simulink model "six_plus_six_AcmsteeringV09_main"  (R2014a)
settings: Solver=FixedStepDiscrete  StartTime=0.0  StopTime=10.0  FixedStep=0.0005  RelTol=1e-3
InitFcn:
  | Veh_Par_wxt
values from neighbouring files (symbols this model uses):
  acc_spdctl = [0 100]    [Veh_Par_wxt.m]
  ag_thr = ecucoder_cal(ag_thr)    [Veh_Par_wxt.m]
  B = 1.8    [Veh_Par_wxt.m]
  bra_em = 100    [Veh_Par_wxt.m]
  bra_pre_gz2 = 100/3    (= 33.3333333333)    [Veh_Par_wxt.m]
  bra_pre_gz34 = 10/3    (= 3.33333333333)    [Veh_Par_wxt.m]
  bra_pre_yd = 10/2    (= 5)    [Veh_Par_wxt.m]
  brakepre_dem_data = [0 1 2 3 4 5 6 7 8 9 10]    [Veh_Par_wxt.m]
  brakeTrq_dem_data = [0 125 251 376 502 627 753 878 1004 1129 1255]    [Veh_Par_wxt.m]
  bratrq_max = 4*1255    (= 5020)    [Veh_Par_wxt.m]
  eff_tran = 0.9    [Veh_Par_wxt.m]
  ESP_switch = ecucoder_cal(ESP_switch)    [Veh_Par_wxt.m]
  G = Mass*g    (= 15696)    [Veh_Par_wxt.m]
  kd1 = ecucoder_cal(kd1)    [Veh_Par_wxt.m]
  kd2 = 0    [Veh_Par_wxt.m]
  ki1 = ecucoder_cal(ki1)    [Veh_Par_wxt.m]
  ki2 = 1    [Veh_Par_wxt.m]
  kp1 = ecucoder_cal(kp1)    [Veh_Par_wxt.m]
  kp2 = 300    [Veh_Par_wxt.m]
  L = L1+L2    (= 2.9)    [Veh_Par_wxt.m]
  premax = 100    [Veh_Par_wxt.m]
  Radius = 0.4572/2    (= 0.2286)    [Veh_Par_wxt.m]
  RC_switch = ecucoder_cal(RC_switch)    [Veh_Par_wxt.m]
  s_opt_yi = 0.15    [Veh_Par_wxt.m]
  s_opt_zhuan = 0.8    [Veh_Par_wxt.m]
  s_opt_zhuan_add = 0.05    [Veh_Par_wxt.m]
  s_opt_zhuan_table = [0.8 0.8 0.3 0.3]    [Veh_Par_wxt.m]
  spd_map_mot = [0 499.85 999.79 1500 2000 2500 3000 3500 4000 4500 4999.8 5999.8]    [Veh_Par_wxt.m]
  spd_spdctl = [0 500]    [Veh_Par_wxt.m]
  speed_thr_park = 5/3.6/Radius*tras_ratio*30/pi    (= 464.143899364)    [Veh_Par_wxt.m]
  TCS_switch = ecucoder_cal(TCS_switch)    [Veh_Par_wxt.m]
  tras_ratio = 8    [Veh_Par_wxt.m]
  trq_map_mot = [70.5 70.012 71.154 65.797 53.917 45.159 38.073 32.685 27.48 17.133 14.949 10.07]    [Veh_Par_wxt.m]
  trqmax_yd = 70.5    [Veh_Par_wxt.m]
  trqmax_zx = 70.5    [Veh_Par_wxt.m]
  trqmaxneg = -70.5    [Veh_Par_wxt.m]
  v_gain = 0.9    [Veh_Par_wxt.m]
  v_table = [0 5 20 100]    [Veh_Par_wxt.m]
  v_thr_park = 5    [Veh_Par_wxt.m]
  zhidong_bianmazhi = [-140000 750000]    [Veh_Par_wxt.m]
  zhidong_down = -140000    [Veh_Par_wxt.m]
  zhidong_up = 750000    [Veh_Par_wxt.m]
  zhidong_youmen = [0 100]    [Veh_Par_wxt.m]
  zhuanxiang_bianmazhi = [-400000 0 400000]    [Veh_Par_wxt.m]
  zhuanxiang_down = -400000    [Veh_Par_wxt.m]
  zhuanxiang_up = 400000    [Veh_Par_wxt.m]
  zhuanxiang_youmen = [-100 0 100]    [Veh_Par_wxt.m]
undefined symbols (not defined in the file or in its folder): ecucoder_acal, guzhang_lf, guzhang_lm, guzhang_lr, guzhang_rf, guzhang_rm, guzhang_rr, myFIS
libraries: simulink x979, ec5744lib x59, fuzblock x2
(part 5 of 26)

== system six_plus_six_AcmsteeringV09_main/Data_input/7/Enabled Subsystem ==
  In2 : Inport
  Enable : EnablePort
  Data Type Conversion{,1..7} (8 alike) : DataTypeConversion
  Demux1 : Demux  Outputs=8
  MATLAB Function : MATLAB Function  TreatAsAtomicUnit=on
  MATLAB Function1 : MATLAB Function  TreatAsAtomicUnit=on
  NorthSpd_Out : Outport
  SkySpd_Out : Outport  Port=2
  wires:
  Demux1/8 -> Data Type Conversion7/1
  Demux1/7 -> Data Type Conversion6/1
  Demux1/6 -> Data Type Conversion5/1
  Demux1/5 -> Data Type Conversion4/1
  MATLAB Function1/1(y) -> SkySpd_Out/1
  MATLAB Function/1(y) -> NorthSpd_Out/1
  Demux1/1 -> Data Type Conversion/1
  Demux1/2 -> Data Type Conversion1/1
  Demux1/3 -> Data Type Conversion2/1
  Demux1/4 -> Data Type Conversion3/1
  In2/1 -> Demux1/1
  Data Type Conversion/1 -> MATLAB Function/1(data1)
  Data Type Conversion2/1 -> MATLAB Function/3(data3)
  Data Type Conversion1/1 -> MATLAB Function/2(data2)
  Data Type Conversion6/1 -> MATLAB Function1/3(data3)
  Data Type Conversion5/1 -> MATLAB Function1/2(data2)
  Data Type Conversion4/1 -> MATLAB Function1/1(data1)
  Data Type Conversion7/1 -> MATLAB Function1/4(data4)
  Data Type Conversion3/1 -> MATLAB Function/4(data4)

== system six_plus_six_AcmsteeringV09_main/Data_input/8/Enabled Subsystem ==
  In2 : Inport
  Enable : EnablePort
  Data Type Conversion{,1..7} (8 alike) : DataTypeConversion
  Demux1 : Demux  Outputs=8
  MATLAB Function : MATLAB Function  TreatAsAtomicUnit=on
  MATLAB Function1 : MATLAB Function  TreatAsAtomicUnit=on
  EastSpd_Out : Outport
  Altitude_Out : Outport  Port=2
  wires:
  In2/1 -> Demux1/1
  Demux1/4 -> Data Type Conversion3/1
  Demux1/3 -> Data Type Conversion2/1
  Demux1/2 -> Data Type Conversion1/1
  Demux1/1 -> Data Type Conversion/1
  MATLAB Function/1(y) -> EastSpd_Out/1
  MATLAB Function1/1(y) -> Altitude_Out/1
  Demux1/5 -> Data Type Conversion4/1
  Demux1/6 -> Data Type Conversion5/1
  Demux1/7 -> Data Type Conversion6/1
  Demux1/8 -> Data Type Conversion7/1
  Data Type Conversion/1 -> MATLAB Function/1(data1)
  Data Type Conversion5/1 -> MATLAB Function1/2(data2)
  Data Type Conversion2/1 -> MATLAB Function/3(data3)
  Data Type Conversion1/1 -> MATLAB Function/2(data2)
  Data Type Conversion7/1 -> MATLAB Function1/4(data4)
  Data Type Conversion4/1 -> MATLAB Function1/1(data1)
  Data Type Conversion6/1 -> MATLAB Function1/3(data3)
  Data Type Conversion3/1 -> MATLAB Function/4(data4)

== system six_plus_six_AcmsteeringV09_main/Data_input/9/Enabled Subsystem ==
  In2 : Inport
  Enable : EnablePort
  Data Type Conversion{,1..7} (8 alike) : DataTypeConversion
  Demux1 : Demux  Outputs=8
  MATLAB Function : MATLAB Function  TreatAsAtomicUnit=on
  MATLAB Function1 : MATLAB Function  TreatAsAtomicUnit=on
  Longitude_Out : Outport
  Latitude_Out : Outport  Port=2
  wires:
  Demux1/8 -> Data Type Conversion7/1
  Demux1/7 -> Data Type Conversion6/1
  Demux1/6 -> Data Type Conversion5/1
  Demux1/5 -> Data Type Conversion4/1
  MATLAB Function1/1(y) -> Latitude_Out/1
  MATLAB Function/1(y) -> Longitude_Out/1
  Demux1/1 -> Data Type Conversion/1
  Demux1/2 -> Data Type Conversion1/1
  Demux1/3 -> Data Type Conversion2/1
  Demux1/4 -> Data Type Conversion3/1
  In2/1 -> Demux1/1
  Data Type Conversion4/1 -> MATLAB Function1/1(data1)
  Data Type Conversion2/1 -> MATLAB Function/3(data3)
  Data Type Conversion1/1 -> MATLAB Function/2(data2)
  Data Type Conversion3/1 -> MATLAB Function/4(data4)
  Data Type Conversion5/1 -> MATLAB Function1/2(data2)
  Data Type Conversion6/1 -> MATLAB Function1/3(data3)
  Data Type Conversion/1 -> MATLAB Function/1(data1)
  Data Type Conversion7/1 -> MATLAB Function1/4(data4)

== system six_plus_six_AcmsteeringV09_main/Data_input/BMS1/BMS1 ==
  input : Inport
  Enable : EnablePort
  BMS1_SOC_Ad : Sum
  BMS1_SOC_Convert : DataTypeConversion  OutDataTypeStr=uint32
  BMS1_SOC_F : Gain  Gain=0.1
  BMS1_SOC_L : simulink/Logic and Bit Operations/Bitwise Operator  logicop=AND  UseBitMask=on  BitMask=65535  BitMaskRealWorld=Stored Integer
  BMS1_SOC_O : Constant  Value=0  OutDataTypeStr=single
  BMS1_SOC_S : ArithShift
  BMS1_SOC_Sub : Subsystem
  BMS1_SOC_sat : Saturate  UpperLimit=1000  LowerLimit=0
  BMS1_SOCcv : DataTypeConversion
  BMS1_SOCinput5_Ad : Sum
  BMS1_SOCinput5_C : Constant  Value=256
  BMS1_SOCinput5_P : Product
  BMS1_Sys_Status1_Ad : Sum
  BMS1_Sys_Status1_Convert : DataTypeConversion  OutDataTypeStr=uint32
  BMS1_Sys_Status1_F : Gain
  BMS1_Sys_Status1_L : simulink/Logic and Bit Operations/Bitwise Operator  logicop=AND  UseBitMask=on  BitMask=255  BitMaskRealWorld=Stored Integer
  BMS1_Sys_Status1_O : Constant  Value=0  OutDataTypeStr=single
  BMS1_Sys_Status1_S : ArithShift
  BMS1_Sys_Status1_Sub : Subsystem
  BMS1_Sys_Status1_sat : Saturate  UpperLimit=255  LowerLimit=0
  BMS1_Sys_Status1cv : DataTypeConversion
  BMS1_Sys_Status2_Ad : Sum
  BMS1_Sys_Status2_Convert : DataTypeConversion  OutDataTypeStr=uint32
  BMS1_Sys_Status2_F : Gain
  BMS1_Sys_Status2_L : simulink/Logic and Bit Operations/Bitwise Operator  logicop=AND  UseBitMask=on  BitMask=255  BitMaskRealWorld=Stored Integer
  BMS1_Sys_Status2_O : Constant  Value=0  OutDataTypeStr=single
  BMS1_Sys_Status2_S : ArithShift
  BMS1_Sys_Status2_Sub : Subsystem
  BMS1_Sys_Status2_sat : Saturate  UpperLimit=255  LowerLimit=0
  BMS1_Sys_Status2cv : DataTypeConversion
  BMS1_TotalCurrent_Ad : Sum
  BMS1_TotalCurrent_Convert : DataTypeConversion  OutDataTypeStr=uint32
  BMS1_TotalCurrent_F : Gain  Gain=0.1
  BMS1_TotalCurrent_L : simulink/Logic and Bit Operations/Bitwise Operator  logicop=AND  UseBitMask=on  BitMask=65535  BitMaskRealWorld=Stored Integer
  BMS1_TotalCurrent_O : Constant  Value=-32000  OutDataTypeStr=single
  BMS1_TotalCurrent_S : ArithShift
  BMS1_TotalCurrent_Sub : Subsystem
  BMS1_TotalCurrent_sat : Saturate  UpperLimit=3353.5  LowerLimit=-32000
  BMS1_TotalCurrentcv : DataTypeConversion
  BMS1_TotalCurrentinput3_Ad : Sum
  BMS1_TotalCurrentinput3_C : Constant  Value=256
  BMS1_TotalCurrentinput3_P : Product
  BMS1_TotalVol_Ad : Sum
  BMS1_TotalVol_Convert : DataTypeConversion  OutDataTypeStr=uint32
  BMS1_TotalVol_F : Gain  Gain=0.1
  BMS1_TotalVol_L : simulink/Logic and Bit Operations/Bitwise Operator  logicop=AND  UseBitMask=on  BitMask=65535  BitMaskRealWorld=Stored Integer
  BMS1_TotalVol_O : Constant  Value=0  OutDataTypeStr=single
  BMS1_TotalVol_S : ArithShift
  BMS1_TotalVol_Sub : Subsystem
  BMS1_TotalVol_sat : Saturate  UpperLimit=6553.5  LowerLimit=0
  BMS1_TotalVolcv : DataTypeConversion
  BMS1_TotalVolinput1_Ad : Sum
  BMS1_TotalVolinput1_C : Constant  Value=256
  BMS1_TotalVolinput1_P : Product
  Demux : Demux  Outputs=8
  BMS1_TotalVol_Out : Outport
  BMS1_TotalCurrent_Out : Outport  Port=2
  BMS1_Sys_Status2_Out : Outport  Port=3
  BMS1_Sys_Status1_Out : Outport  Port=4
  BMS1_SOC_Out : Outport  Port=5
  wires:
  BMS1_TotalVol_F/1 -> BMS1_TotalVol_Ad/1
  BMS1_TotalVol_O/1 -> BMS1_TotalVol_Ad/2
  BMS1_TotalVol_Ad/1 -> BMS1_TotalVol_sat/1
  BMS1_TotalVol_sat/1 -> BMS1_TotalVol_Out/1
  Demux/1 -> BMS1_TotalVolinput1_P/1
  BMS1_TotalVolinput1_C/1 -> BMS1_TotalVolinput1_P/2
  BMS1_TotalVolinput1_P/1 -> BMS1_TotalVolinput1_Ad/1
  Demux/2 -> BMS1_TotalVolinput1_Ad/2
  BMS1_TotalVolinput1_Ad/1 -> BMS1_TotalVol_Sub/1(In1)
  BMS1_TotalVol_Sub/1(Out1) -> BMS1_TotalVol_Convert/1
  BMS1_TotalVol_Convert/1 -> BMS1_TotalVol_L/1
  BMS1_TotalVol_L/1 -> BMS1_TotalVol_S/1
  BMS1_TotalVol_S/1 -> BMS1_TotalVolcv/1
  BMS1_TotalVolcv/1 -> BMS1_TotalVol_F/1
  BMS1_TotalCurrent_F/1 -> BMS1_TotalCurrent_Ad/1
  BMS1_TotalCurrent_O/1 -> BMS1_TotalCurrent_Ad/2
  BMS1_TotalCurrent_Ad/1 -> BMS1_TotalCurrent_sat/1
  BMS1_TotalCurrent_sat/1 -> BMS1_TotalCurrent_Out/1
  Demux/3 -> BMS1_TotalCurrentinput3_P/1
  BMS1_TotalCurrentinput3_C/1 -> BMS1_TotalCurrentinput3_P/2
  BMS1_TotalCurrentinput3_P/1 -> BMS1_TotalCurrentinput3_Ad/1
  Demux/4 -> BMS1_TotalCurrentinput3_Ad/2
  BMS1_TotalCurrentinput3_Ad/1 -> BMS1_TotalCurrent_Sub/1(In1)
  BMS1_TotalCurrent_Sub/1(Out1) -> BMS1_TotalCurrent_Convert/1
  BMS1_TotalCurrent_Convert/1 -> BMS1_TotalCurrent_L/1
  BMS1_TotalCurrent_L/1 -> BMS1_TotalCurrent_S/1
  BMS1_TotalCurrent_S/1 -> BMS1_TotalCurrentcv/1
  BMS1_TotalCurrentcv/1 -> BMS1_TotalCurrent_F/1
  BMS1_Sys_Status2_F/1 -> BMS1_Sys_Status2_Ad/1
  BMS1_Sys_Status2_O/1 -> BMS1_Sys_Status2_Ad/2
  BMS1_Sys_Status2_Ad/1 -> BMS1_Sys_Status2_sat/1
  BMS1_Sys_Status2_sat/1 -> BMS1_Sys_Status2_Out/1
  Demux/8 -> BMS1_Sys_Status2_Sub/1(In1)
  BMS1_Sys_Status2_Sub/1(Out1) -> BMS1_Sys_Status2_Convert/1
  BMS1_Sys_Status2_Convert/1 -> BMS1_Sys_Status2_L/1
  BMS1_Sys_Status2_L/1 -> BMS1_Sys_Status2_S/1
  BMS1_Sys_Status2_S/1 -> BMS1_Sys_Status2cv/1
  BMS1_Sys_Status2cv/1 -> BMS1_Sys_Status2_F/1
  BMS1_Sys_Status1_F/1 -> BMS1_Sys_Status1_Ad/1
  BMS1_Sys_Status1_O/1 -> BMS1_Sys_Status1_Ad/2
  BMS1_Sys_Status1_Ad/1 -> BMS1_Sys_Status1_sat/1
  BMS1_Sys_Status1_sat/1 -> BMS1_Sys_Status1_Out/1
  Demux/7 -> BMS1_Sys_Status1_Sub/1(In1)
  BMS1_Sys_Status1_Sub/1(Out1) -> BMS1_Sys_Status1_Convert/1
  BMS1_Sys_Status1_Convert/1 -> BMS1_Sys_Status1_L/1
  BMS1_Sys_Status1_L/1 -> BMS1_Sys_Status1_S/1
  BMS1_Sys_Status1_S/1 -> BMS1_Sys_Status1cv/1
  BMS1_Sys_Status1cv/1 -> BMS1_Sys_Status1_F/1
  BMS1_SOC_F/1 -> BMS1_SOC_Ad/1
  BMS1_SOC_O/1 -> BMS1_SOC_Ad/2
  BMS1_SOC_Ad/1 -> BMS1_SOC_sat/1
  BMS1_SOC_sat/1 -> BMS1_SOC_Out/1
  Demux/5 -> BMS1_SOCinput5_P/1
  BMS1_SOCinput5_C/1 -> BMS1_SOCinput5_P/2
  BMS1_SOCinput5_P/1 -> BMS1_SOCinput5_Ad/1
  Demux/6 -> BMS1_SOCinput5_Ad/2
  BMS1_SOCinput5_Ad/1 -> BMS1_SOC_Sub/1(In1)
  BMS1_SOC_Sub/1(Out1) -> BMS1_SOC_Convert/1
  BMS1_SOC_Convert/1 -> BMS1_SOC_L/1
  BMS1_SOC_L/1 -> BMS1_SOC_S/1
  BMS1_SOC_S/1 -> BMS1_SOCcv/1
  BMS1_SOCcv/1 -> BMS1_SOC_F/1
  input/1 -> Demux/1

== system six_plus_six_AcmsteeringV09_main/Data_input/BMS1-2/BMS1 ==
  input : Inport
  Enable : EnablePort
  BMS1_SOC_Ad : Sum
  BMS1_SOC_Convert : DataTypeConversion  OutDataTypeStr=uint32
  BMS1_SOC_F : Gain  Gain=0.1
  BMS1_SOC_L : simulink/Logic and Bit Operations/Bitwise Operator  logicop=AND  UseBitMask=on  BitMask=65535  BitMaskRealWorld=Stored Integer
  BMS1_SOC_O : Constant  Value=0  OutDataTypeStr=single
  BMS1_SOC_S : ArithShift
  BMS1_SOC_Sub : Subsystem
  BMS1_SOC_sat : Saturate  UpperLimit=1000  LowerLimit=0
  BMS1_SOCcv : DataTypeConversion
  BMS1_SOCinput5_Ad : Sum
  BMS1_SOCinput5_C : Constant  Value=256
  BMS1_SOCinput5_P : Product
  BMS1_Sys_Status1_Ad : Sum
  BMS1_Sys_Status1_Convert : DataTypeConversion  OutDataTypeStr=uint32
  BMS1_Sys_Status1_F : Gain
  BMS1_Sys_Status1_L : simulink/Logic and Bit Operations/Bitwise Operator  logicop=AND  UseBitMask=on  BitMask=255  BitMaskRealWorld=Stored Integer
  BMS1_Sys_Status1_O : Constant  Value=0  OutDataTypeStr=single
  BMS1_Sys_Status1_S : ArithShift
  BMS1_Sys_Status1_Sub : Subsystem
  BMS1_Sys_Status1_sat : Saturate  UpperLimit=255  LowerLimit=0
  BMS1_Sys_Status1cv : DataTypeConversion
  BMS1_Sys_Status2_Ad : Sum
  BMS1_Sys_Status2_Convert : DataTypeConversion  OutDataTypeStr=uint32
  BMS1_Sys_Status2_F : Gain
  BMS1_Sys_Status2_L : simulink/Logic and Bit Operations/Bitwise Operator  logicop=AND  UseBitMask=on  BitMask=255  BitMaskRealWorld=Stored Integer
  BMS1_Sys_Status2_O : Constant  Value=0  OutDataTypeStr=single
  BMS1_Sys_Status2_S : ArithShift
  BMS1_Sys_Status2_Sub : Subsystem
  BMS1_Sys_Status2_sat : Saturate  UpperLimit=255  LowerLimit=0
  BMS1_Sys_Status2cv : DataTypeConversion
  BMS1_TotalCurrent_Ad : Sum
  BMS1_TotalCurrent_Convert : DataTypeConversion  OutDataTypeStr=uint32
  BMS1_TotalCurrent_F : Gain  Gain=0.1
  BMS1_TotalCurrent_L : simulink/Logic and Bit Operations/Bitwise Operator  logicop=AND  UseBitMask=on  BitMask=65535  BitMaskRealWorld=Stored Integer
  BMS1_TotalCurrent_O : Constant  Value=-32000  OutDataTypeStr=single
  BMS1_TotalCurrent_S : ArithShift
  BMS1_TotalCurrent_Sub : Subsystem
  BMS1_TotalCurrent_sat : Saturate  UpperLimit=3353.5  LowerLimit=-32000
  BMS1_TotalCurrentcv : DataTypeConversion
  BMS1_TotalCurrentinput3_Ad : Sum
  BMS1_TotalCurrentinput3_C : Constant  Value=256
  BMS1_TotalCurrentinput3_P : Product
  BMS1_TotalVol_Ad : Sum
  BMS1_TotalVol_Convert : DataTypeConversion  OutDataTypeStr=uint32
  BMS1_TotalVol_F : Gain  Gain=0.1
  BMS1_TotalVol_L : simulink/Logic and Bit Operations/Bitwise Operator  logicop=AND  UseBitMask=on  BitMask=65535  BitMaskRealWorld=Stored Integer
  BMS1_TotalVol_O : Constant  Value=0  OutDataTypeStr=single
  BMS1_TotalVol_S : ArithShift
  BMS1_TotalVol_Sub : Subsystem
  BMS1_TotalVol_sat : Saturate  UpperLimit=6553.5  LowerLimit=0
  BMS1_TotalVolcv : DataTypeConversion
  BMS1_TotalVolinput1_Ad : Sum
  BMS1_TotalVolinput1_C : Constant  Value=256
  BMS1_TotalVolinput1_P : Product
  Demux : Demux  Outputs=8
  BMS1_TotalVol_Out : Outport
  BMS1_TotalCurrent_Out : Outport  Port=2
  BMS1_Sys_Status2_Out : Outport  Port=3
  BMS1_Sys_Status1_Out : Outport  Port=4
  BMS1_SOC_Out : Outport  Port=5
  wires:
  BMS1_TotalVol_F/1 -> BMS1_TotalVol_Ad/1
  BMS1_TotalVol_O/1 -> BMS1_TotalVol_Ad/2
  BMS1_TotalVol_Ad/1 -> BMS1_TotalVol_sat/1
  BMS1_TotalVol_sat/1 -> BMS1_TotalVol_Out/1
  Demux/1 -> BMS1_TotalVolinput1_P/1
  BMS1_TotalVolinput1_C/1 -> BMS1_TotalVolinput1_P/2
  BMS1_TotalVolinput1_P/1 -> BMS1_TotalVolinput1_Ad/1
  Demux/2 -> BMS1_TotalVolinput1_Ad/2
  BMS1_TotalVolinput1_Ad/1 -> BMS1_TotalVol_Sub/1(In1)
  BMS1_TotalVol_Sub/1(Out1) -> BMS1_TotalVol_Convert/1
  BMS1_TotalVol_Convert/1 -> BMS1_TotalVol_L/1
  BMS1_TotalVol_L/1 -> BMS1_TotalVol_S/1
  BMS1_TotalVol_S/1 -> BMS1_TotalVolcv/1
  BMS1_TotalVolcv/1 -> BMS1_TotalVol_F/1
  BMS1_TotalCurrent_F/1 -> BMS1_TotalCurrent_Ad/1
  BMS1_TotalCurrent_O/1 -> BMS1_TotalCurrent_Ad/2
  BMS1_TotalCurrent_Ad/1 -> BMS1_TotalCurrent_sat/1
  BMS1_TotalCurrent_sat/1 -> BMS1_TotalCurrent_Out/1
  Demux/3 -> BMS1_TotalCurrentinput3_P/1
  BMS1_TotalCurrentinput3_C/1 -> BMS1_TotalCurrentinput3_P/2
  BMS1_TotalCurrentinput3_P/1 -> BMS1_TotalCurrentinput3_Ad/1
  Demux/4 -> BMS1_TotalCurrentinput3_Ad/2
  BMS1_TotalCurrentinput3_Ad/1 -> BMS1_TotalCurrent_Sub/1(In1)
  BMS1_TotalCurrent_Sub/1(Out1) -> BMS1_TotalCurrent_Convert/1
  BMS1_TotalCurrent_Convert/1 -> BMS1_TotalCurrent_L/1
  BMS1_TotalCurrent_L/1 -> BMS1_TotalCurrent_S/1
  BMS1_TotalCurrent_S/1 -> BMS1_TotalCurrentcv/1
  BMS1_TotalCurrentcv/1 -> BMS1_TotalCurrent_F/1
  BMS1_Sys_Status2_F/1 -> BMS1_Sys_Status2_Ad/1
  BMS1_Sys_Status2_O/1 -> BMS1_Sys_Status2_Ad/2
  BMS1_Sys_Status2_Ad/1 -> BMS1_Sys_Status2_sat/1
  BMS1_Sys_Status2_sat/1 -> BMS1_Sys_Status2_Out/1
  Demux/8 -> BMS1_Sys_Status2_Sub/1(In1)
  BMS1_Sys_Status2_Sub/1(Out1) -> BMS1_Sys_Status2_Convert/1
  BMS1_Sys_Status2_Convert/1 -> BMS1_Sys_Status2_L/1
  BMS1_Sys_Status2_L/1 -> BMS1_Sys_Status2_S/1
  BMS1_Sys_Status2_S/1 -> BMS1_Sys_Status2cv/1
  BMS1_Sys_Status2cv/1 -> BMS1_Sys_Status2_F/1
  BMS1_Sys_Status1_F/1 -> BMS1_Sys_Status1_Ad/1
  BMS1_Sys_Status1_O/1 -> BMS1_Sys_Status1_Ad/2
  BMS1_Sys_Status1_Ad/1 -> BMS1_Sys_Status1_sat/1
  BMS1_Sys_Status1_sat/1 -> BMS1_Sys_Status1_Out/1
  Demux/7 -> BMS1_Sys_Status1_Sub/1(In1)
  BMS1_Sys_Status1_Sub/1(Out1) -> BMS1_Sys_Status1_Convert/1
  BMS1_Sys_Status1_Convert/1 -> BMS1_Sys_Status1_L/1
  BMS1_Sys_Status1_L/1 -> BMS1_Sys_Status1_S/1
  BMS1_Sys_Status1_S/1 -> BMS1_Sys_Status1cv/1
  BMS1_Sys_Status1cv/1 -> BMS1_Sys_Status1_F/1
  BMS1_SOC_F/1 -> BMS1_SOC_Ad/1
  BMS1_SOC_O/1 -> BMS1_SOC_Ad/2
  BMS1_SOC_Ad/1 -> BMS1_SOC_sat/1
  BMS1_SOC_sat/1 -> BMS1_SOC_Out/1
  Demux/5 -> BMS1_SOCinput5_P/1
  BMS1_SOCinput5_C/1 -> BMS1_SOCinput5_P/2
  BMS1_SOCinput5_P/1 -> BMS1_SOCinput5_Ad/1
  Demux/6 -> BMS1_SOCinput5_Ad/2
  BMS1_SOCinput5_Ad/1 -> BMS1_SOC_Sub/1(In1)
  BMS1_SOC_Sub/1(Out1) -> BMS1_SOC_Convert/1
  BMS1_SOC_Convert/1 -> BMS1_SOC_L/1
  BMS1_SOC_L/1 -> BMS1_SOC_S/1
  BMS1_SOC_S/1 -> BMS1_SOCcv/1
  BMS1_SOCcv/1 -> BMS1_SOC_F/1
  input/1 -> Demux/1

== system six_plus_six_AcmsteeringV09_main/Data_input/BMS1_1/BMS1 ==
  input : Inport
  Enable : EnablePort
  BMS1_SOC_Ad : Sum
  BMS1_SOC_Convert : DataTypeConversion  OutDataTypeStr=uint32
  BMS1_SOC_F : Gain  Gain=0.1
  BMS1_SOC_L : simulink/Logic and Bit Operations/Bitwise Operator  logicop=AND  UseBitMask=on  BitMask=65535  BitMaskRealWorld=Stored Integer
  BMS1_SOC_O : Constant  Value=0  OutDataTypeStr=single
  BMS1_SOC_S : ArithShift
  BMS1_SOC_Sub : Subsystem
  BMS1_SOC_sat : Saturate  UpperLimit=1000  LowerLimit=0
  BMS1_SOCcv : DataTypeConversion
  BMS1_SOCinput5_Ad : Sum
  BMS1_SOCinput5_C : Constant  Value=256
  BMS1_SOCinput5_P : Product
  BMS1_Sys_Status1_Ad : Sum
  BMS1_Sys_Status1_Convert : DataTypeConversion  OutDataTypeStr=uint32
  BMS1_Sys_Status1_F : Gain
  BMS1_Sys_Status1_L : simulink/Logic and Bit Operations/Bitwise Operator  logicop=AND  UseBitMask=on  BitMask=255  BitMaskRealWorld=Stored Integer
  BMS1_Sys_Status1_O : Constant  Value=0  OutDataTypeStr=single
  BMS1_Sys_Status1_S : ArithShift
  BMS1_Sys_Status1_Sub : Subsystem
  BMS1_Sys_Status1_sat : Saturate  UpperLimit=255  LowerLimit=0
  BMS1_Sys_Status1cv : DataTypeConversion
  BMS1_Sys_Status2_Ad : Sum
  BMS1_Sys_Status2_Convert : DataTypeConversion  OutDataTypeStr=uint32
  BMS1_Sys_Status2_F : Gain
  BMS1_Sys_Status2_L : simulink/Logic and Bit Operations/Bitwise Operator  logicop=AND  UseBitMask=on  BitMask=255  BitMaskRealWorld=Stored Integer
  BMS1_Sys_Status2_O : Constant  Value=0  OutDataTypeStr=single
  BMS1_Sys_Status2_S : ArithShift
  BMS1_Sys_Status2_Sub : Subsystem
  BMS1_Sys_Status2_sat : Saturate  UpperLimit=255  LowerLimit=0
  BMS1_Sys_Status2cv : DataTypeConversion
  BMS1_TotalCurrent_Ad : Sum
  BMS1_TotalCurrent_Convert : DataTypeConversion  OutDataTypeStr=uint32
  BMS1_TotalCurrent_F : Gain  Gain=0.1
  BMS1_TotalCurrent_L : simulink/Logic and Bit Operations/Bitwise Operator  logicop=AND  UseBitMask=on  BitMask=65535  BitMaskRealWorld=Stored Integer
  BMS1_TotalCurrent_O : Constant  Value=-32000  OutDataTypeStr=single
  BMS1_TotalCurrent_S : ArithShift
  BMS1_TotalCurrent_Sub : Subsystem
  BMS1_TotalCurrent_sat : Saturate  UpperLimit=3353.5  LowerLimit=-32000
  BMS1_TotalCurrentcv : DataTypeConversion
  BMS1_TotalCurrentinput3_Ad : Sum
  BMS1_TotalCurrentinput3_C : Constant  Value=256
  BMS1_TotalCurrentinput3_P : Product
  BMS1_TotalVol_Ad : Sum
  BMS1_TotalVol_Convert : DataTypeConversion  OutDataTypeStr=uint32
  BMS1_TotalVol_F : Gain  Gain=0.1
  BMS1_TotalVol_L : simulink/Logic and Bit Operations/Bitwise Operator  logicop=AND  UseBitMask=on  BitMask=65535  BitMaskRealWorld=Stored Integer
  BMS1_TotalVol_O : Constant  Value=0  OutDataTypeStr=single
  BMS1_TotalVol_S : ArithShift
  BMS1_TotalVol_Sub : Subsystem
  BMS1_TotalVol_sat : Saturate  UpperLimit=6553.5  LowerLimit=0
  BMS1_TotalVolcv : DataTypeConversion
  BMS1_TotalVolinput1_Ad : Sum
  BMS1_TotalVolinput1_C : Constant  Value=256
  BMS1_TotalVolinput1_P : Product
  Demux : Demux  Outputs=8
  BMS1_TotalVol_Out : Outport
  BMS1_TotalCurrent_Out : Outport  Port=2
  BMS1_Sys_Status2_Out : Outport  Port=3
  BMS1_Sys_Status1_Out : Outport  Port=4
  BMS1_SOC_Out : Outport  Port=5
  wires:
  BMS1_TotalVol_F/1 -> BMS1_TotalVol_Ad/1
  BMS1_TotalVol_O/1 -> BMS1_TotalVol_Ad/2
  BMS1_TotalVol_Ad/1 -> BMS1_TotalVol_sat/1
  BMS1_TotalVol_sat/1 -> BMS1_TotalVol_Out/1
  Demux/1 -> BMS1_TotalVolinput1_P/1
  BMS1_TotalVolinput1_C/1 -> BMS1_TotalVolinput1_P/2
  BMS1_TotalVolinput1_P/1 -> BMS1_TotalVolinput1_Ad/1
  Demux/2 -> BMS1_TotalVolinput1_Ad/2
  BMS1_TotalVolinput1_Ad/1 -> BMS1_TotalVol_Sub/1(In1)
  BMS1_TotalVol_Sub/1(Out1) -> BMS1_TotalVol_Convert/1
  BMS1_TotalVol_Convert/1 -> BMS1_TotalVol_L/1
  BMS1_TotalVol_L/1 -> BMS1_TotalVol_S/1
  BMS1_TotalVol_S/1 -> BMS1_TotalVolcv/1
  BMS1_TotalVolcv/1 -> BMS1_TotalVol_F/1
  BMS1_TotalCurrent_F/1 -> BMS1_TotalCurrent_Ad/1
  BMS1_TotalCurrent_O/1 -> BMS1_TotalCurrent_Ad/2
  BMS1_TotalCurrent_Ad/1 -> BMS1_TotalCurrent_sat/1
  BMS1_TotalCurrent_sat/1 -> BMS1_TotalCurrent_Out/1
  Demux/3 -> BMS1_TotalCurrentinput3_P/1
  BMS1_TotalCurrentinput3_C/1 -> BMS1_TotalCurrentinput3_P/2
  BMS1_TotalCurrentinput3_P/1 -> BMS1_TotalCurrentinput3_Ad/1
  Demux/4 -> BMS1_TotalCurrentinput3_Ad/2
  BMS1_TotalCurrentinput3_Ad/1 -> BMS1_TotalCurrent_Sub/1(In1)
  BMS1_TotalCurrent_Sub/1(Out1) -> BMS1_TotalCurrent_Convert/1
  BMS1_TotalCurrent_Convert/1 -> BMS1_TotalCurrent_L/1
  BMS1_TotalCurrent_L/1 -> BMS1_TotalCurrent_S/1
  BMS1_TotalCurrent_S/1 -> BMS1_TotalCurrentcv/1
  BMS1_TotalCurrentcv/1 -> BMS1_TotalCurrent_F/1
  BMS1_Sys_Status2_F/1 -> BMS1_Sys_Status2_Ad/1
  BMS1_Sys_Status2_O/1 -> BMS1_Sys_Status2_Ad/2
  BMS1_Sys_Status2_Ad/1 -> BMS1_Sys_Status2_sat/1
  BMS1_Sys_Status2_sat/1 -> BMS1_Sys_Status2_Out/1
  Demux/8 -> BMS1_Sys_Status2_Sub/1(In1)
  BMS1_Sys_Status2_Sub/1(Out1) -> BMS1_Sys_Status2_Convert/1
  BMS1_Sys_Status2_Convert/1 -> BMS1_Sys_Status2_L/1
  BMS1_Sys_Status2_L/1 -> BMS1_Sys_Status2_S/1
  BMS1_Sys_Status2_S/1 -> BMS1_Sys_Status2cv/1
  BMS1_Sys_Status2cv/1 -> BMS1_Sys_Status2_F/1
  BMS1_Sys_Status1_F/1 -> BMS1_Sys_Status1_Ad/1
  BMS1_Sys_Status1_O/1 -> BMS1_Sys_Status1_Ad/2
  BMS1_Sys_Status1_Ad/1 -> BMS1_Sys_Status1_sat/1
  BMS1_Sys_Status1_sat/1 -> BMS1_Sys_Status1_Out/1
  Demux/7 -> BMS1_Sys_Status1_Sub/1(In1)
  BMS1_Sys_Status1_Sub/1(Out1) -> BMS1_Sys_Status1_Convert/1
  BMS1_Sys_Status1_Convert/1 -> BMS1_Sys_Status1_L/1
  BMS1_Sys_Status1_L/1 -> BMS1_Sys_Status1_S/1
  BMS1_Sys_Status1_S/1 -> BMS1_Sys_Status1cv/1
  BMS1_Sys_Status1cv/1 -> BMS1_Sys_Status1_F/1
  BMS1_SOC_F/1 -> BMS1_SOC_Ad/1
  BMS1_SOC_O/1 -> BMS1_SOC_Ad/2
  BMS1_SOC_Ad/1 -> BMS1_SOC_sat/1
  BMS1_SOC_sat/1 -> BMS1_SOC_Out/1
  Demux/5 -> BMS1_SOCinput5_P/1
  BMS1_SOCinput5_C/1 -> BMS1_SOCinput5_P/2
  BMS1_SOCinput5_P/1 -> BMS1_SOCinput5_Ad/1
  Demux/6 -> BMS1_SOCinput5_Ad/2
  BMS1_SOCinput5_Ad/1 -> BMS1_SOC_Sub/1(In1)
  BMS1_SOC_Sub/1(Out1) -> BMS1_SOC_Convert/1
  BMS1_SOC_Convert/1 -> BMS1_SOC_L/1
  BMS1_SOC_L/1 -> BMS1_SOC_S/1
  BMS1_SOC_S/1 -> BMS1_SOCcv/1
  BMS1_SOCcv/1 -> BMS1_SOC_F/1
  input/1 -> Demux/1

== system six_plus_six_AcmsteeringV09_main/Data_input/BMS2/BMS2 ==
  input : Inport
  Enable : EnablePort
  BMS2_HighSingleVol_Ad : Sum
  BMS2_HighSingleVol_Convert : DataTypeConversion  OutDataTypeStr=uint32
  BMS2_HighSingleVol_F : Gain
  BMS2_HighSingleVol_L : simulink/Logic and Bit Operations/Bitwise Operator  logicop=AND  UseBitMask=on  BitMask=65535  BitMaskRealWorld=Stored Integer
  BMS2_HighSingleVol_O : Constant  Value=0  OutDataTypeStr=single
  BMS2_HighSingleVol_S : ArithShift
  BMS2_HighSingleVol_Sub : Subsystem
  BMS2_HighSingleVol_sat : Saturate  UpperLimit=10  LowerLimit=0
  BMS2_HighSingleVolcv : DataTypeConversion
  BMS2_HighSingleVolinput1_Ad : Sum
  BMS2_HighSingleVolinput1_C : Constant  Value=256
  BMS2_HighSingleVolinput1_P : Product
  BMS2_LowSingleVol_Ad : Sum
  BMS2_LowSingleVol_Convert : DataTypeConversion  OutDataTypeStr=uint32
  BMS2_LowSingleVol_F : Gain
  BMS2_LowSingleVol_L : simulink/Logic and Bit Operations/Bitwise Operator  logicop=AND  UseBitMask=on  BitMask=65535  BitMaskRealWorld=Stored Integer
  BMS2_LowSingleVol_O : Constant  Value=0  OutDataTypeStr=single
  BMS2_LowSingleVol_S : ArithShift
  BMS2_LowSingleVol_Sub : Subsystem
  BMS2_LowSingleVol_sat : Saturate  UpperLimit=65535  LowerLimit=0
  BMS2_LowSingleVolcv : DataTypeConversion
  BMS2_LowSingleVolinput3_Ad : Sum
  BMS2_LowSingleVolinput3_C : Constant  Value=256
  BMS2_LowSingleVolinput3_P : Product
  Demux : Demux  Outputs=8
  BMS2_LowSingleVol_Out : Outport
  BMS2_HighSingleVol_Out : Outport  Port=2
  wires:
  BMS2_LowSingleVol_F/1 -> BMS2_LowSingleVol_Ad/1
  BMS2_LowSingleVol_O/1 -> BMS2_LowSingleVol_Ad/2
  BMS2_LowSingleVol_Ad/1 -> BMS2_LowSingleVol_sat/1
  BMS2_LowSingleVol_sat/1 -> BMS2_LowSingleVol_Out/1
  Demux/3 -> BMS2_LowSingleVolinput3_P/1
  BMS2_LowSingleVolinput3_C/1 -> BMS2_LowSingleVolinput3_P/2
  BMS2_LowSingleVolinput3_P/1 -> BMS2_LowSingleVolinput3_Ad/1
  Demux/4 -> BMS2_LowSingleVolinput3_Ad/2
  BMS2_LowSingleVolinput3_Ad/1 -> BMS2_LowSingleVol_Sub/1(In1)
  BMS2_LowSingleVol_Sub/1(Out1) -> BMS2_LowSingleVol_Convert/1
  BMS2_LowSingleVol_Convert/1 -> BMS2_LowSingleVol_L/1
  BMS2_LowSingleVol_L/1 -> BMS2_LowSingleVol_S/1
  BMS2_LowSingleVol_S/1 -> BMS2_LowSingleVolcv/1
  BMS2_LowSingleVolcv/1 -> BMS2_LowSingleVol_F/1
  BMS2_HighSingleVol_F/1 -> BMS2_HighSingleVol_Ad/1
  BMS2_HighSingleVol_O/1 -> BMS2_HighSingleVol_Ad/2
  BMS2_HighSingleVol_Ad/1 -> BMS2_HighSingleVol_sat/1
  BMS2_HighSingleVol_sat/1 -> BMS2_HighSingleVol_Out/1
  Demux/1 -> BMS2_HighSingleVolinput1_P/1
  BMS2_HighSingleVolinput1_C/1 -> BMS2_HighSingleVolinput1_P/2
  BMS2_HighSingleVolinput1_P/1 -> BMS2_HighSingleVolinput1_Ad/1
  Demux/2 -> BMS2_HighSingleVolinput1_Ad/2
  BMS2_HighSingleVolinput1_Ad/1 -> BMS2_HighSingleVol_Sub/1(In1)
  BMS2_HighSingleVol_Sub/1(Out1) -> BMS2_HighSingleVol_Convert/1
  BMS2_HighSingleVol_Convert/1 -> BMS2_HighSingleVol_L/1
  BMS2_HighSingleVol_L/1 -> BMS2_HighSingleVol_S/1
  BMS2_HighSingleVol_S/1 -> BMS2_HighSingleVolcv/1
  BMS2_HighSingleVolcv/1 -> BMS2_HighSingleVol_F/1
  input/1 -> Demux/1

== system six_plus_six_AcmsteeringV09_main/Data_input/BMS2_1/BMS2 ==
  input : Inport
  Enable : EnablePort
  BMS2_HighSingleVol_Ad : Sum
  BMS2_HighSingleVol_Convert : DataTypeConversion  OutDataTypeStr=uint32
  BMS2_HighSingleVol_F : Gain
  BMS2_HighSingleVol_L : simulink/Logic and Bit Operations/Bitwise Operator  logicop=AND  UseBitMask=on  BitMask=65535  BitMaskRealWorld=Stored Integer
  BMS2_HighSingleVol_O : Constant  Value=0  OutDataTypeStr=single
  BMS2_HighSingleVol_S : ArithShift
  BMS2_HighSingleVol_Sub : Subsystem
  BMS2_HighSingleVol_sat : Saturate  UpperLimit=10  LowerLimit=0
  BMS2_HighSingleVolcv : DataTypeConversion
  BMS2_HighSingleVolinput1_Ad : Sum
  BMS2_HighSingleVolinput1_C : Constant  Value=256
  BMS2_HighSingleVolinput1_P : Product
  BMS2_LowSingleVol_Ad : Sum
  BMS2_LowSingleVol_Convert : DataTypeConversion  OutDataTypeStr=uint32
  BMS2_LowSingleVol_F : Gain
  BMS2_LowSingleVol_L : simulink/Logic and Bit Operations/Bitwise Operator  logicop=AND  UseBitMask=on  BitMask=65535  BitMaskRealWorld=Stored Integer
  BMS2_LowSingleVol_O : Constant  Value=0  OutDataTypeStr=single
  BMS2_LowSingleVol_S : ArithShift
  BMS2_LowSingleVol_Sub : Subsystem
  BMS2_LowSingleVol_sat : Saturate  UpperLimit=65535  LowerLimit=0
  BMS2_LowSingleVolcv : DataTypeConversion
  BMS2_LowSingleVolinput3_Ad : Sum
  BMS2_LowSingleVolinput3_C : Constant  Value=256
  BMS2_LowSingleVolinput3_P : Product
  Demux : Demux  Outputs=8
  BMS2_LowSingleVol_Out : Outport
  BMS2_HighSingleVol_Out : Outport  Port=2
  wires:
  BMS2_LowSingleVol_F/1 -> BMS2_LowSingleVol_Ad/1
  BMS2_LowSingleVol_O/1 -> BMS2_LowSingleVol_Ad/2
  BMS2_LowSingleVol_Ad/1 -> BMS2_LowSingleVol_sat/1
  BMS2_LowSingleVol_sat/1 -> BMS2_LowSingleVol_Out/1
  Demux/3 -> BMS2_LowSingleVolinput3_P/1
  BMS2_LowSingleVolinput3_C/1 -> BMS2_LowSingleVolinput3_P/2
  BMS2_LowSingleVolinput3_P/1 -> BMS2_LowSingleVolinput3_Ad/1
  Demux/4 -> BMS2_LowSingleVolinput3_Ad/2
  BMS2_LowSingleVolinput3_Ad/1 -> BMS2_LowSingleVol_Sub/1(In1)
  BMS2_LowSingleVol_Sub/1(Out1) -> BMS2_LowSingleVol_Convert/1
  BMS2_LowSingleVol_Convert/1 -> BMS2_LowSingleVol_L/1
  BMS2_LowSingleVol_L/1 -> BMS2_LowSingleVol_S/1
  BMS2_LowSingleVol_S/1 -> BMS2_LowSingleVolcv/1
  BMS2_LowSingleVolcv/1 -> BMS2_LowSingleVol_F/1
  BMS2_HighSingleVol_F/1 -> BMS2_HighSingleVol_Ad/1
  BMS2_HighSingleVol_O/1 -> BMS2_HighSingleVol_Ad/2
  BMS2_HighSingleVol_Ad/1 -> BMS2_HighSingleVol_sat/1
  BMS2_HighSingleVol_sat/1 -> BMS2_HighSingleVol_Out/1
  Demux/1 -> BMS2_HighSingleVolinput1_P/1
  BMS2_HighSingleVolinput1_C/1 -> BMS2_HighSingleVolinput1_P/2
  BMS2_HighSingleVolinput1_P/1 -> BMS2_HighSingleVolinput1_Ad/1
  Demux/2 -> BMS2_HighSingleVolinput1_Ad/2
  BMS2_HighSingleVolinput1_Ad/1 -> BMS2_HighSingleVol_Sub/1(In1)
  BMS2_HighSingleVol_Sub/1(Out1) -> BMS2_HighSingleVol_Convert/1
  BMS2_HighSingleVol_Convert/1 -> BMS2_HighSingleVol_L/1
  BMS2_HighSingleVol_L/1 -> BMS2_HighSingleVol_S/1
  BMS2_HighSingleVol_S/1 -> BMS2_HighSingleVolcv/1
  BMS2_HighSingleVolcv/1 -> BMS2_HighSingleVol_F/1
  input/1 -> Demux/1

== system six_plus_six_AcmsteeringV09_main/Data_input/BMS2_2/BMS2 ==
  input : Inport
  Enable : EnablePort
  BMS2_HighSingleVol_Ad : Sum
  BMS2_HighSingleVol_Convert : DataTypeConversion  OutDataTypeStr=uint32
  BMS2_HighSingleVol_F : Gain
  BMS2_HighSingleVol_L : simulink/Logic and Bit Operations/Bitwise Operator  logicop=AND  UseBitMask=on  BitMask=65535  BitMaskRealWorld=Stored Integer
  BMS2_HighSingleVol_O : Constant  Value=0  OutDataTypeStr=single
  BMS2_HighSingleVol_S : ArithShift
  BMS2_HighSingleVol_Sub : Subsystem
  BMS2_HighSingleVol_sat : Saturate  UpperLimit=10  LowerLimit=0
  BMS2_HighSingleVolcv : DataTypeConversion
  BMS2_HighSingleVolinput1_Ad : Sum
  BMS2_HighSingleVolinput1_C : Constant  Value=256
  BMS2_HighSingleVolinput1_P : Product
  BMS2_LowSingleVol_Ad : Sum
  BMS2_LowSingleVol_Convert : DataTypeConversion  OutDataTypeStr=uint32
  BMS2_LowSingleVol_F : Gain
  BMS2_LowSingleVol_L : simulink/Logic and Bit Operations/Bitwise Operator  logicop=AND  UseBitMask=on  BitMask=65535  BitMaskRealWorld=Stored Integer
  BMS2_LowSingleVol_O : Constant  Value=0  OutDataTypeStr=single
  BMS2_LowSingleVol_S : ArithShift
  BMS2_LowSingleVol_Sub : Subsystem
  BMS2_LowSingleVol_sat : Saturate  UpperLimit=65535  LowerLimit=0
  BMS2_LowSingleVolcv : DataTypeConversion
  BMS2_LowSingleVolinput3_Ad : Sum
  BMS2_LowSingleVolinput3_C : Constant  Value=256
  BMS2_LowSingleVolinput3_P : Product
  Demux : Demux  Outputs=8
  BMS2_LowSingleVol_Out : Outport
  BMS2_HighSingleVol_Out : Outport  Port=2
  wires:
  BMS2_LowSingleVol_F/1 -> BMS2_LowSingleVol_Ad/1
  BMS2_LowSingleVol_O/1 -> BMS2_LowSingleVol_Ad/2
  BMS2_LowSingleVol_Ad/1 -> BMS2_LowSingleVol_sat/1
  BMS2_LowSingleVol_sat/1 -> BMS2_LowSingleVol_Out/1
  Demux/3 -> BMS2_LowSingleVolinput3_P/1
  BMS2_LowSingleVolinput3_C/1 -> BMS2_LowSingleVolinput3_P/2
  BMS2_LowSingleVolinput3_P/1 -> BMS2_LowSingleVolinput3_Ad/1
  Demux/4 -> BMS2_LowSingleVolinput3_Ad/2
  BMS2_LowSingleVolinput3_Ad/1 -> BMS2_LowSingleVol_Sub/1(In1)
  BMS2_LowSingleVol_Sub/1(Out1) -> BMS2_LowSingleVol_Convert/1
  BMS2_LowSingleVol_Convert/1 -> BMS2_LowSingleVol_L/1
  BMS2_LowSingleVol_L/1 -> BMS2_LowSingleVol_S/1
  BMS2_LowSingleVol_S/1 -> BMS2_LowSingleVolcv/1
  BMS2_LowSingleVolcv/1 -> BMS2_LowSingleVol_F/1
  BMS2_HighSingleVol_F/1 -> BMS2_HighSingleVol_Ad/1
  BMS2_HighSingleVol_O/1 -> BMS2_HighSingleVol_Ad/2
  BMS2_HighSingleVol_Ad/1 -> BMS2_HighSingleVol_sat/1
  BMS2_HighSingleVol_sat/1 -> BMS2_HighSingleVol_Out/1
  Demux/1 -> BMS2_HighSingleVolinput1_P/1
  BMS2_HighSingleVolinput1_C/1 -> BMS2_HighSingleVolinput1_P/2
  BMS2_HighSingleVolinput1_P/1 -> BMS2_HighSingleVolinput1_Ad/1
  Demux/2 -> BMS2_HighSingleVolinput1_Ad/2
  BMS2_HighSingleVolinput1_Ad/1 -> BMS2_HighSingleVol_Sub/1(In1)
  BMS2_HighSingleVol_Sub/1(Out1) -> BMS2_HighSingleVol_Convert/1
  BMS2_HighSingleVol_Convert/1 -> BMS2_HighSingleVol_L/1
  BMS2_HighSingleVol_L/1 -> BMS2_HighSingleVol_S/1
  BMS2_HighSingleVol_S/1 -> BMS2_HighSingleVolcv/1
  BMS2_HighSingleVolcv/1 -> BMS2_HighSingleVol_F/1
  input/1 -> Demux/1

== system six_plus_six_AcmsteeringV09_main/Data_input/BMS3/BMS3 ==
  input : Inport
  Enable : EnablePort
  BMS3_HighTemperature_Ad : Sum
  BMS3_HighTemperature_Convert : DataTypeConversion  OutDataTypeStr=uint32
  BMS3_HighTemperature_F : Gain
  BMS3_HighTemperature_L : simulink/Logic and Bit Operations/Bitwise Operator  logicop=AND  UseBitMask=on  BitMask=255  BitMaskRealWorld=Stored Integer
  BMS3_HighTemperature_O : Constant  Value=-40  OutDataTypeStr=single
  BMS3_HighTemperature_S : ArithShift
  BMS3_HighTemperature_Sub : Subsystem
  BMS3_HighTemperature_sat : Saturate  UpperLimit=210  LowerLimit=-40
  BMS3_HighTemperaturecv : DataTypeConversion
  BMS3_LowTemperature_Ad : Sum
  BMS3_LowTemperature_Convert : DataTypeConversion  OutDataTypeStr=uint32
  BMS3_LowTemperature_F : Gain
  BMS3_LowTemperature_L : simulink/Logic and Bit Operations/Bitwise Operator  logicop=AND  UseBitMask=on  BitMask=255  BitMaskRealWorld=Stored Integer
  BMS3_LowTemperature_O : Constant  Value=-40  OutDataTypeStr=single
  BMS3_LowTemperature_S : ArithShift
  BMS3_LowTemperature_Sub : Subsystem
  BMS3_LowTemperature_sat : Saturate  UpperLimit=210  LowerLimit=-40
  BMS3_LowTemperaturecv : DataTypeConversion
  Demux : Demux  Outputs=8
  BMS3_LowTemperature_Out : Outport
  BMS3_HighTemperature_Out : Outport  Port=2
  wires:
  BMS3_LowTemperature_F/1 -> BMS3_LowTemperature_Ad/1
  BMS3_LowTemperature_O/1 -> BMS3_LowTemperature_Ad/2
  BMS3_LowTemperature_Ad/1 -> BMS3_LowTemperature_sat/1
  BMS3_LowTemperature_sat/1 -> BMS3_LowTemperature_Out/1
  Demux/3 -> BMS3_LowTemperature_Sub/1(In1)
  BMS3_LowTemperature_Sub/1(Out1) -> BMS3_LowTemperature_Convert/1
  BMS3_LowTemperature_Convert/1 -> BMS3_LowTemperature_L/1
  BMS3_LowTemperature_L/1 -> BMS3_LowTemperature_S/1
  BMS3_LowTemperature_S/1 -> BMS3_LowTemperaturecv/1
  BMS3_LowTemperaturecv/1 -> BMS3_LowTemperature_F/1
  BMS3_HighTemperature_F/1 -> BMS3_HighTemperature_Ad/1
  BMS3_HighTemperature_O/1 -> BMS3_HighTemperature_Ad/2
  BMS3_HighTemperature_Ad/1 -> BMS3_HighTemperature_sat/1
  BMS3_HighTemperature_sat/1 -> BMS3_HighTemperature_Out/1
  Demux/1 -> BMS3_HighTemperature_Sub/1(In1)
  BMS3_HighTemperature_Sub/1(Out1) -> BMS3_HighTemperature_Convert/1
  BMS3_HighTemperature_Convert/1 -> BMS3_HighTemperature_L/1
  BMS3_HighTemperature_L/1 -> BMS3_HighTemperature_S/1
  BMS3_HighTemperature_S/1 -> BMS3_HighTemperaturecv/1
  BMS3_HighTemperaturecv/1 -> BMS3_HighTemperature_F/1
  input/1 -> Demux/1

== system six_plus_six_AcmsteeringV09_main/Data_input/BMS3_1/BMS3 ==
  input : Inport
  Enable : EnablePort
  BMS3_HighTemperature_Ad : Sum
  BMS3_HighTemperature_Convert : DataTypeConversion  OutDataTypeStr=uint32
  BMS3_HighTemperature_F : Gain
  BMS3_HighTemperature_L : simulink/Logic and Bit Operations/Bitwise Operator  logicop=AND  UseBitMask=on  BitMask=255  BitMaskRealWorld=Stored Integer
  BMS3_HighTemperature_O : Constant  Value=-40  OutDataTypeStr=single
  BMS3_HighTemperature_S : ArithShift
  BMS3_HighTemperature_Sub : Subsystem
  BMS3_HighTemperature_sat : Saturate  UpperLimit=210  LowerLimit=-40
  BMS3_HighTemperaturecv : DataTypeConversion
  BMS3_LowTemperature_Ad : Sum
  BMS3_LowTemperature_Convert : DataTypeConversion  OutDataTypeStr=uint32
  BMS3_LowTemperature_F : Gain
  BMS3_LowTemperature_L : simulink/Logic and Bit Operations/Bitwise Operator  logicop=AND  UseBitMask=on  BitMask=255  BitMaskRealWorld=Stored Integer
  BMS3_LowTemperature_O : Constant  Value=-40  OutDataTypeStr=single
  BMS3_LowTemperature_S : ArithShift
  BMS3_LowTemperature_Sub : Subsystem
  BMS3_LowTemperature_sat : Saturate  UpperLimit=210  LowerLimit=-40
  BMS3_LowTemperaturecv : DataTypeConversion
  Demux : Demux  Outputs=8
  BMS3_LowTemperature_Out : Outport
  BMS3_HighTemperature_Out : Outport  Port=2
  wires:
  BMS3_LowTemperature_F/1 -> BMS3_LowTemperature_Ad/1
  BMS3_LowTemperature_O/1 -> BMS3_LowTemperature_Ad/2
  BMS3_LowTemperature_Ad/1 -> BMS3_LowTemperature_sat/1
  BMS3_LowTemperature_sat/1 -> BMS3_LowTemperature_Out/1
  Demux/3 -> BMS3_LowTemperature_Sub/1(In1)
  BMS3_LowTemperature_Sub/1(Out1) -> BMS3_LowTemperature_Convert/1
  BMS3_LowTemperature_Convert/1 -> BMS3_LowTemperature_L/1
  BMS3_LowTemperature_L/1 -> BMS3_LowTemperature_S/1
  BMS3_LowTemperature_S/1 -> BMS3_LowTemperaturecv/1
  BMS3_LowTemperaturecv/1 -> BMS3_LowTemperature_F/1
  BMS3_HighTemperature_F/1 -> BMS3_HighTemperature_Ad/1
  BMS3_HighTemperature_O/1 -> BMS3_HighTemperature_Ad/2
  BMS3_HighTemperature_Ad/1 -> BMS3_HighTemperature_sat/1
  BMS3_HighTemperature_sat/1 -> BMS3_HighTemperature_Out/1
  Demux/1 -> BMS3_HighTemperature_Sub/1(In1)
  BMS3_HighTemperature_Sub/1(Out1) -> BMS3_HighTemperature_Convert/1
  BMS3_HighTemperature_Convert/1 -> BMS3_HighTemperature_L/1
  BMS3_HighTemperature_L/1 -> BMS3_HighTemperature_S/1
  BMS3_HighTemperature_S/1 -> BMS3_HighTemperaturecv/1
  BMS3_HighTemperaturecv/1 -> BMS3_HighTemperature_F/1
  input/1 -> Demux/1

== system six_plus_six_AcmsteeringV09_main/Data_input/BMS3_2/BMS3 ==
  input : Inport
  Enable : EnablePort
  BMS3_HighTemperature_Ad : Sum
  BMS3_HighTemperature_Convert : DataTypeConversion  OutDataTypeStr=uint32
  BMS3_HighTemperature_F : Gain
  BMS3_HighTemperature_L : simulink/Logic and Bit Operations/Bitwise Operator  logicop=AND  UseBitMask=on  BitMask=255  BitMaskRealWorld=Stored Integer
  BMS3_HighTemperature_O : Constant  Value=-40  OutDataTypeStr=single
  BMS3_HighTemperature_S : ArithShift
  BMS3_HighTemperature_Sub : Subsystem
  BMS3_HighTemperature_sat : Saturate  UpperLimit=210  LowerLimit=-40
  BMS3_HighTemperaturecv : DataTypeConversion
  BMS3_LowTemperature_Ad : Sum
  BMS3_LowTemperature_Convert : DataTypeConversion  OutDataTypeStr=uint32
  BMS3_LowTemperature_F : Gain
  BMS3_LowTemperature_L : simulink/Logic and Bit Operations/Bitwise Operator  logicop=AND  UseBitMask=on  BitMask=255  BitMaskRealWorld=Stored Integer
  BMS3_LowTemperature_O : Constant  Value=-40  OutDataTypeStr=single
  BMS3_LowTemperature_S : ArithShift
  BMS3_LowTemperature_Sub : Subsystem
  BMS3_LowTemperature_sat : Saturate  UpperLimit=210  LowerLimit=-40
  BMS3_LowTemperaturecv : DataTypeConversion
  Demux : Demux  Outputs=8
  BMS3_LowTemperature_Out : Outport
  BMS3_HighTemperature_Out : Outport  Port=2
  wires:
  BMS3_LowTemperature_F/1 -> BMS3_LowTemperature_Ad/1
  BMS3_LowTemperature_O/1 -> BMS3_LowTemperature_Ad/2
  BMS3_LowTemperature_Ad/1 -> BMS3_LowTemperature_sat/1
  BMS3_LowTemperature_sat/1 -> BMS3_LowTemperature_Out/1
  Demux/3 -> BMS3_LowTemperature_Sub/1(In1)
  BMS3_LowTemperature_Sub/1(Out1) -> BMS3_LowTemperature_Convert/1
  BMS3_LowTemperature_Convert/1 -> BMS3_LowTemperature_L/1
  BMS3_LowTemperature_L/1 -> BMS3_LowTemperature_S/1
  BMS3_LowTemperature_S/1 -> BMS3_LowTemperaturecv/1
  BMS3_LowTemperaturecv/1 -> BMS3_LowTemperature_F/1
  BMS3_HighTemperature_F/1 -> BMS3_HighTemperature_Ad/1
  BMS3_HighTemperature_O/1 -> BMS3_HighTemperature_Ad/2
  BMS3_HighTemperature_Ad/1 -> BMS3_HighTemperature_sat/1
  BMS3_HighTemperature_sat/1 -> BMS3_HighTemperature_Out/1
  Demux/1 -> BMS3_HighTemperature_Sub/1(In1)
  BMS3_HighTemperature_Sub/1(Out1) -> BMS3_HighTemperature_Convert/1
  BMS3_HighTemperature_Convert/1 -> BMS3_HighTemperature_L/1
  BMS3_HighTemperature_L/1 -> BMS3_HighTemperature_S/1
  BMS3_HighTemperature_S/1 -> BMS3_HighTemperaturecv/1
  BMS3_HighTemperaturecv/1 -> BMS3_HighTemperature_F/1
  input/1 -> Demux/1

== system six_plus_six_AcmsteeringV09_main/Data_input/BMS4/BMS4 ==
  input : Inport
  Enable : EnablePort
  BMS4_InputVolACC_Ad : Sum
  BMS4_InputVolACC_Convert : DataTypeConversion  OutDataTypeStr=uint32
  BMS4_InputVolACC_F : Gain  Gain=0.1
  BMS4_InputVolACC_L : simulink/Logic and Bit Operations/Bitwise Operator  logicop=AND  UseBitMask=on  BitMask=65535  BitMaskRealWorld=Stored Integer
  BMS4_InputVolACC_O : Constant  Value=0  OutDataTypeStr=single
  BMS4_InputVolACC_S : ArithShift
  BMS4_InputVolACC_Sub : Subsystem
  BMS4_InputVolACC_sat : Saturate  UpperLimit=6553.5  LowerLimit=0
  BMS4_InputVolACCcv : DataTypeConversion
  BMS4_InputVolACCinput2_Ad : Sum
  BMS4_InputVolACCinput2_C : Constant  Value=256
  BMS4_InputVolACCinput2_P : Product
  BMS4_InputVolCHG_Ad : Sum
  BMS4_InputVolCHG_Convert : DataTypeConversion  OutDataTypeStr=uint32
  BMS4_InputVolCHG_F : Gain  Gain=0.1
  BMS4_InputVolCHG_L : simulink/Logic and Bit Operations/Bitwise Operator  logicop=AND  UseBitMask=on  BitMask=65535  BitMaskRealWorld=Stored Integer
  BMS4_InputVolCHG_O : Constant  Value=0  OutDataTypeStr=single
  BMS4_InputVolCHG_S : ArithShift
  BMS4_InputVolCHG_Sub : Subsystem
  BMS4_InputVolCHG_sat : Saturate  UpperLimit=6553.5  LowerLimit=0
  BMS4_InputVolCHGcv : DataTypeConversion
  BMS4_InputVolCHGinput6_Ad : Sum
  BMS4_InputVolCHGinput6_C : Constant  Value=256
  BMS4_InputVolCHGinput6_P : Product
  BMS4_InputVolKEYON_Ad : Sum
  BMS4_InputVolKEYON_Convert : DataTypeConversion  OutDataTypeStr=uint32
  BMS4_InputVolKEYON_F : Gain  Gain=0.1
  BMS4_InputVolKEYON_L : simulink/Logic and Bit Operations/Bitwise Operator  logicop=AND  UseBitMask=on  BitMask=65535  BitMaskRealWorld=Stored Integer
  BMS4_InputVolKEYON_O : Constant  Value=0  OutDataTypeStr=single
  BMS4_InputVolKEYON_S : ArithShift
  BMS4_InputVolKEYON_Sub : Subsystem
  BMS4_InputVolKEYON_sat : Saturate  UpperLimit=6553.5  LowerLimit=0
  BMS4_InputVolKEYONcv : DataTypeConversion
  BMS4_InputVolKEYONinput4_Ad : Sum
  BMS4_InputVolKEYONinput4_C : Constant  Value=256
  BMS4_InputVolKEYONinput4_P : Product
  BMS4_Sys_Status3_Ad : Sum
  BMS4_Sys_Status3_Convert : DataTypeConversion  OutDataTypeStr=uint32
  BMS4_Sys_Status3_F : Gain
  BMS4_Sys_Status3_L : simulink/Logic and Bit Operations/Bitwise Operator  logicop=AND  UseBitMask=on  BitMask=255  BitMaskRealWorld=Stored Integer
  BMS4_Sys_Status3_O : Constant  Value=0  OutDataTypeStr=single
  BMS4_Sys_Status3_S : ArithShift
  BMS4_Sys_Status3_Sub : Subsystem
  BMS4_Sys_Status3_sat : Saturate  UpperLimit=255  LowerLimit=0
  BMS4_Sys_Status3cv : DataTypeConversion
  Demux : Demux  Outputs=8
  BMS4_Sys_Status3_Out : Outport
  BMS4_InputVolKEYON_Out : Outport  Port=2
  BMS4_InputVolCHG_Out : Outport  Port=3
  BMS4_InputVolACC_Out : Outport  Port=4
  wires:
  BMS4_Sys_Status3_F/1 -> BMS4_Sys_Status3_Ad/1
  BMS4_Sys_Status3_O/1 -> BMS4_Sys_Status3_Ad/2
  BMS4_Sys_Status3_Ad/1 -> BMS4_Sys_Status3_sat/1
  BMS4_Sys_Status3_sat/1 -> BMS4_Sys_Status3_Out/1
  Demux/1 -> BMS4_Sys_Status3_Sub/1(In1)
  BMS4_Sys_Status3_Sub/1(Out1) -> BMS4_Sys_Status3_Convert/1
  BMS4_Sys_Status3_Convert/1 -> BMS4_Sys_Status3_L/1
  BMS4_Sys_Status3_L/1 -> BMS4_Sys_Status3_S/1
  BMS4_Sys_Status3_S/1 -> BMS4_Sys_Status3cv/1
  BMS4_Sys_Status3cv/1 -> BMS4_Sys_Status3_F/1
  BMS4_InputVolKEYON_F/1 -> BMS4_InputVolKEYON_Ad/1
  BMS4_InputVolKEYON_O/1 -> BMS4_InputVolKEYON_Ad/2
  BMS4_InputVolKEYON_Ad/1 -> BMS4_InputVolKEYON_sat/1
  BMS4_InputVolKEYON_sat/1 -> BMS4_InputVolKEYON_Out/1
  Demux/4 -> BMS4_InputVolKEYONinput4_P/1
  BMS4_InputVolKEYONinput4_C/1 -> BMS4_InputVolKEYONinput4_P/2
  BMS4_InputVolKEYONinput4_P/1 -> BMS4_InputVolKEYONinput4_Ad/1
  Demux/5 -> BMS4_InputVolKEYONinput4_Ad/2
  BMS4_InputVolKEYONinput4_Ad/1 -> BMS4_InputVolKEYON_Sub/1(In1)
  BMS4_InputVolKEYON_Sub/1(Out1) -> BMS4_InputVolKEYON_Convert/1
  BMS4_InputVolKEYON_Convert/1 -> BMS4_InputVolKEYON_L/1
  BMS4_InputVolKEYON_L/1 -> BMS4_InputVolKEYON_S/1
  BMS4_InputVolKEYON_S/1 -> BMS4_InputVolKEYONcv/1
  BMS4_InputVolKEYONcv/1 -> BMS4_InputVolKEYON_F/1
  BMS4_InputVolCHG_F/1 -> BMS4_InputVolCHG_Ad/1
  BMS4_InputVolCHG_O/1 -> BMS4_InputVolCHG_Ad/2
  BMS4_InputVolCHG_Ad/1 -> BMS4_InputVolCHG_sat/1
  BMS4_InputVolCHG_sat/1 -> BMS4_InputVolCHG_Out/1
  Demux/6 -> BMS4_InputVolCHGinput6_P/1
  BMS4_InputVolCHGinput6_C/1 -> BMS4_InputVolCHGinput6_P/2
  BMS4_InputVolCHGinput6_P/1 -> BMS4_InputVolCHGinput6_Ad/1
  Demux/7 -> BMS4_InputVolCHGinput6_Ad/2
  BMS4_InputVolCHGinput6_Ad/1 -> BMS4_InputVolCHG_Sub/1(In1)
  BMS4_InputVolCHG_Sub/1(Out1) -> BMS4_InputVolCHG_Convert/1
  BMS4_InputVolCHG_Convert/1 -> BMS4_InputVolCHG_L/1
  BMS4_InputVolCHG_L/1 -> BMS4_InputVolCHG_S/1
  BMS4_InputVolCHG_S/1 -> BMS4_InputVolCHGcv/1
  BMS4_InputVolCHGcv/1 -> BMS4_InputVolCHG_F/1
  BMS4_InputVolACC_F/1 -> BMS4_InputVolACC_Ad/1
  BMS4_InputVolACC_O/1 -> BMS4_InputVolACC_Ad/2
  BMS4_InputVolACC_Ad/1 -> BMS4_InputVolACC_sat/1
  BMS4_InputVolACC_sat/1 -> BMS4_InputVolACC_Out/1
  Demux/2 -> BMS4_InputVolACCinput2_P/1
  BMS4_InputVolACCinput2_C/1 -> BMS4_InputVolACCinput2_P/2
  BMS4_InputVolACCinput2_P/1 -> BMS4_InputVolACCinput2_Ad/1
  Demux/3 -> BMS4_InputVolACCinput2_Ad/2
  BMS4_InputVolACCinput2_Ad/1 -> BMS4_InputVolACC_Sub/1(In1)
  BMS4_InputVolACC_Sub/1(Out1) -> BMS4_InputVolACC_Convert/1
  BMS4_InputVolACC_Convert/1 -> BMS4_InputVolACC_L/1
  BMS4_InputVolACC_L/1 -> BMS4_InputVolACC_S/1
  BMS4_InputVolACC_S/1 -> BMS4_InputVolACCcv/1
  BMS4_InputVolACCcv/1 -> BMS4_InputVolACC_F/1
  input/1 -> Demux/1

== matlab function six_plus_six_AcmsteeringV09_main/MainControl/mode_control/center_steer/center_steer/HeartBeat3 ==
  data: life_pre input; life output
function life = fcn(life_pre)
%#codegen
life=single(life_pre+1);
if life>255
    life=single(0);
end
end

== matlab function six_plus_six_AcmsteeringV09_main/MainControl/mode_control/emergency_stop/emergency_stop/HeartBeat ==
  data: life_pre input; life output
function life = fcn(life_pre)
%#codegen
life=single(life_pre+1);
if life>255
    life=single(0);
end
end

== matlab function six_plus_six_AcmsteeringV09_main/MainControl/mode_control/neutral/neutral/HeartBeat4 ==
  data: life_pre input; life output
function life = fcn(life_pre)
%#codegen
life=single(life_pre+1);
if life>255
    life=single(0);
end
end

== matlab function six_plus_six_AcmsteeringV09_main/MainControl/mode_control/forward/forward/Drive/驱动防滑控制TCS/直行TCS/直行/MATLAB Function2 ==
  data: s_act_rf input; flag_rf output; s_opt_zhuan input; s_opt_zhuan_add input; flag_rf_pre input int8
function flag_rf = fcn(s_act_rf,s_opt_zhuan,s_opt_zhuan_add,flag_rf_pre)
%#codegen
if s_act_rf>s_opt_zhuan+s_opt_zhuan_add
    flag_rf=int8(1);
elseif s_act_rf<s_opt_zhuan
    flag_rf =int8(0);
else
    flag_rf=int8(flag_rf_pre);
end
end

== matlab function six_plus_six_AcmsteeringV09_main/Subsystem/MATLAB Function ==
  data: data_1 input; data output; data_2 input; zero output; position_4 output; position_3 output; position_2 output; position_1 output
function [data,zero,position_4,position_3,position_2,position_1] = motec_write(data_1,data_2)
if  data_1<150
    if (mod(data_1,6)<3)
    data=6;
    else
    data=7;
    end
    zero=hex2dec('00');
    position_1=hex2dec('00');
    position_2=hex2dec('00');
    position_3=hex2dec('00');
    position_4=hex2dec('00');  
else
    if (mod(data_1,2)==0)
        data=15;
        zero=hex2dec('00');
    else
        zero=hex2dec('00');
        data=95;    
    end
%Negative numbers are represented with the Two's Complement
       data_2=double(data_2);
       if data_2<0
       data_2= 2^32+data_2;
       end
%Find the 4 bytes
       position_1= floor( data_2/(2^24) );
       remainder1     = floor( mod( data_2,(2^24) ) );
       position_2= floor( remainder1/(2^16) );
       remainder2     = floor( mod( remainder1,(2^16) ) );
       position_3= floor( remainder2/(2^8) );
       position_4= floor( mod( remainder2,(2^8) ) );
 
end

== matlab function six_plus_six_AcmsteeringV09_main/MainControl/mode_control/Park/park/HeartBeat5 ==
  data: life_pre input; life output
function life = fcn(life_pre)
%#codegen
life=single(life_pre+1);
if life>255
    life=single(0);
end
end
